simulink model "e1_2"  (R2022a)
settings: Solver=VariableStepAuto  StartTime=0.0  StopTime=50  FixedStep=0.1  MaxStep=0.1  RelTol=1e-3  AbsTol=1e-6
settings Model: Creator=lenovo  LastModifiedBy=18075
settings SolverCC: AlgebraicLoopSolver=TrustRegion
settings DebuggingCC: UnconnectedInputMsg=warning  UnconnectedOutputMsg=warning  UnconnectedLineMsg=warning  SFMachineParentedDataDiag=warning
settings RTWCC: DLArmComputeVersion=19.05

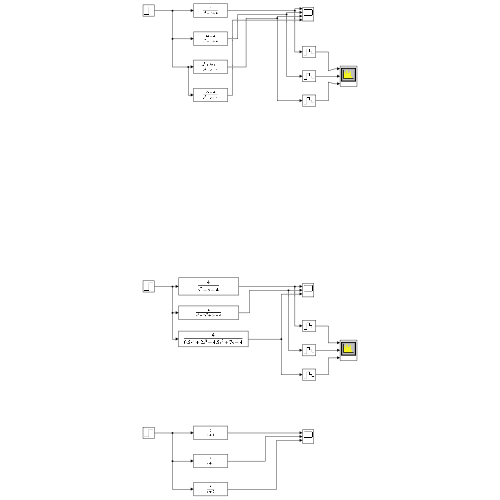
[thumbnail: Simulink's stored preview of the top-level diagram]
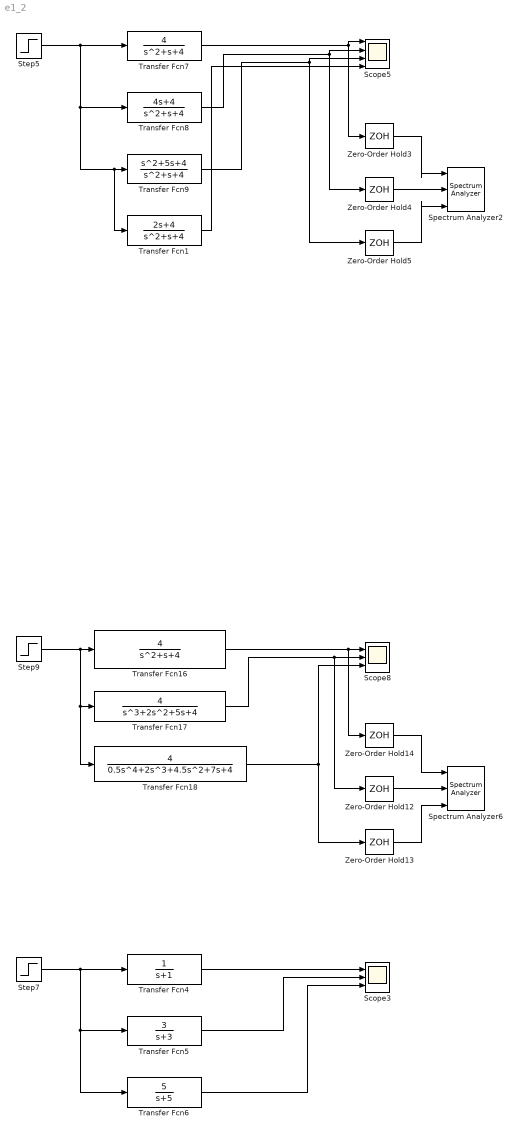
== system e1_2 ==
  Scope3 : Scope  NumInputPorts=3
  Scope5 : Scope  NumInputPorts=4
  Scope8 : Scope  NumInputPorts=3
  Spectrum Analyzer2 : SpectrumAnalyzer  NumInputPorts=3
  Spectrum Analyzer6 : SpectrumAnalyzer  NumInputPorts=3
  Step5 : Step  Time=0  SampleTime=0
  Step7 : Step  Time=0  SampleTime=0
  Step9 : Step  Time=0  SampleTime=0
  Transfer Fcn1 : TransferFcn  Numerator=[2 4]  Denominator=[1 1 4]
  Transfer Fcn16 : TransferFcn  Numerator=[4]  Denominator=[1 1 4]
  Transfer Fcn17 : TransferFcn  Numerator=[4]  Denominator=[1 2 5 4]
  Transfer Fcn18 : TransferFcn  Numerator=[4]  Denominator=[0.5 2 4.5 7 4]
  Transfer Fcn4 : TransferFcn  Denominator=[1 1]
  Transfer Fcn5 : TransferFcn  Numerator=[3]  Denominator=[1 3]
  Transfer Fcn6 : TransferFcn  Numerator=[5]  Denominator=[1 5]
  Transfer Fcn7 : TransferFcn  Numerator=[4]  Denominator=[1 1 4]
  Transfer Fcn8 : TransferFcn  Numerator=[4 4]  Denominator=[1 1 4]
  Transfer Fcn9 : TransferFcn  Numerator=[1 5 4]  Denominator=[1 1 4]
  Zero-Order Hold{3..5,12..14} (6 alike) : ZeroOrderHold  SampleTime=0.01
  wires:
  Transfer Fcn5/1 -> Scope3/2
  Transfer Fcn4/1 -> Scope3/1
  Step7/1 -> Transfer Fcn6/1, Transfer Fcn5/1, Transfer Fcn4/1
  Transfer Fcn6/1 -> Scope3/3
  Step5/1 -> Transfer Fcn1/1, Transfer Fcn9/1, Transfer Fcn8/1, Transfer Fcn7/1
  Transfer Fcn8/1 -> Scope5/2, Zero-Order Hold4/1
  Transfer Fcn7/1 -> Zero-Order Hold3/1, Scope5/1
  Transfer Fcn9/1 -> Zero-Order Hold5/1, Scope5/3
  Zero-Order Hold4/1 -> Spectrum Analyzer2/2
  Zero-Order Hold3/1 -> Spectrum Analyzer2/1
  Zero-Order Hold5/1 -> Spectrum Analyzer2/3
  Step9/1 -> Transfer Fcn16/1, Transfer Fcn18/1, Transfer Fcn17/1
  Transfer Fcn17/1 -> Zero-Order Hold12/1, Scope8/2
  Transfer Fcn16/1 -> Scope8/1, Zero-Order Hold14/1
  Zero-Order Hold14/1 -> Spectrum Analyzer6/1
  Zero-Order Hold13/1 -> Spectrum Analyzer6/3
  Transfer Fcn18/1 -> Scope8/3, Zero-Order Hold13/1
  Zero-Order Hold12/1 -> Spectrum Analyzer6/2
  Transfer Fcn1/1 -> Scope5/4
